simulink model "WTmodel"  (R2016b)
settings: Solver=VariableStepAuto  StartTime=0.0  StopTime=10.0  RelTol=1e-3
values from neighbouring files (symbols this model uses):
  Kb = 56.6    [B2B_SM_wC_data_fromCC_WT.m]
undefined symbols (not defined in the file or in its folder): VPoptpu, wPrefpu
settings Model: Creator=peiyuan  LastModifiedBy=peiyuan

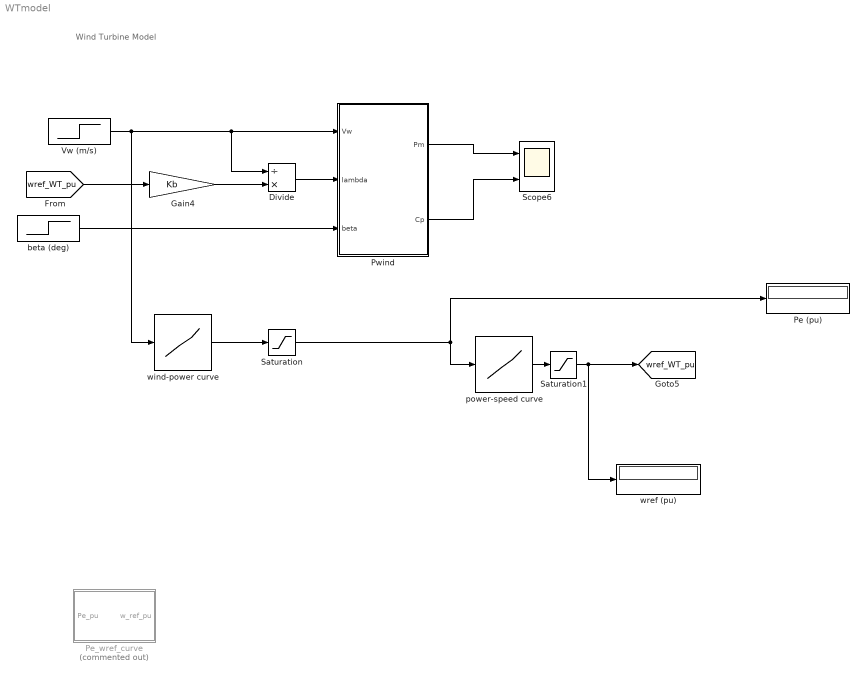
== system WTmodel ==
  note: Wind Turbine Model
  Divide : Product  Inputs=/*
  Gain4 : Gain  Gain=Kb
  Pe (pu) : Display
      settings: Format=bank
  Pe_wref_curve : Subsystem  Commented=on
  Pwind : MATLAB Function  TreatAsAtomicUnit=on
  Saturation : Saturate  UpperLimit=1  LowerLimit=0
  Saturation1 : Saturate  UpperLimit=1.2  LowerLimit=0.1
  Scope6 : Scope  NumInputPorts=2
  "Vw (m/s) " : Step  Time=5  Before=9  After=15  SampleTime=0
  beta (deg) : Step  Time=5  After=11.47  SampleTime=0
  power-speed curve : Lookup_n-D  NumberOfTableDimensions=1  BreakpointsForDimension1=wPrefpu(:,2)  Table=wPrefpu(:,1)  InternalRulePriority=Speed  RndMeth=Simplest  InputSameDT=on
  wind-power curve : Lookup_n-D  NumberOfTableDimensions=1  BreakpointsForDimension1=VPoptpu(:,1)  Table=VPoptpu(:,2)  InternalRulePriority=Speed  RndMeth=Simplest  InputSameDT=on
  wref (pu) : Display
      settings: Format=bank
  tag scope: wref_WT_pu=global
  wires:
  "Vw (m/s) "/1 -> wind-power curve/1, Pwind/1(Vw), Divide/1
  Divide/1 -> Pwind/2(lambda)
  Gain4/1 -> Divide/2
  beta (deg)/1 -> Pwind/3(beta)
  [wref_WT_pu] -> Gain4/1
  Pwind/1(Pm) -> Scope6/1
  Pwind/2(Cp) -> Scope6/2
  wind-power curve/1 -> Saturation/1
  power-speed curve/1 -> Saturation1/1
  Saturation/1 -> power-speed curve/1, Pe (pu)/1
  Saturation1/1 -> wref (pu)/1, [wref_WT_pu]

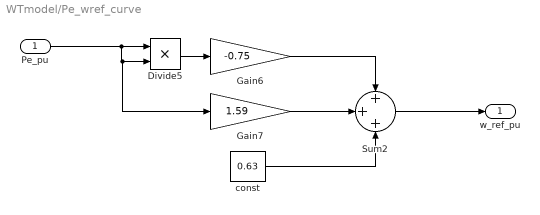
== system WTmodel/Pe_wref_curve ==
  Pe_pu : Inport
  Divide5 : Product  Inputs=**
  Gain6 : Gain  Gain=-0.75
  Gain7 : Gain  Gain=1.59
  Sum2 : Sum  Inputs=+++
  const : Constant  Value=0.63
  w_ref_pu : Outport
  wires:
  Gain7/1 -> Sum2/2
  Gain6/1 -> Sum2/1
  Divide5/1 -> Gain6/1
  Pe_pu/1 -> Gain7/1, Divide5/2, Divide5/1
  const/1 -> Sum2/3
  Sum2/1 -> w_ref_pu/1

== matlab function WTmodel/Pwind ==
  data: Vw input; Pm output; lambda input; beta input; Cp output
function [Pm,Cp] = Pwind(Vw,lambda,beta)

%% Inputs
% Vm
% beta: Pitch angle
% lambda: Tip speed ratio

%% Outputs
% Pm: Mechanical power output
% Cp: aerodynamic efficiency

%% Cp calculation: valid for lambda within (3,15)

alpha=[-4.1909e-1  2.1808e-1  -1.2406e-2  -1.3365e-4   1.1524e-5
       -6.7606e-2  6.0405e-2  -1.3934e-2   1.0683e-3  -2.3895e-5
        1.5727e-2 -1.0996e-2   2.1495e-3  -1.4855e-4   2.7937e-6
       -8.6018e-4  5.7051e-4  -1.0479e-4   5.9924e-6  -8.9194e-8
        1.4787e-5 -9.4839e-6   1.6167e-6  -7.1535e-8   4.9686e-10];

% Size of alpha
sz=size(alpha);
rw=sz(1);
cl=sz(2);

% calculate Cp
y=0;

for kk=1:rw
    
    for jj=1:cl
        
        y=y+alpha(kk,jj)*(beta^(kk-1))*(lambda^(jj-1));
        
    end
end
% Cp=min(max(y,-0.05),0.5173);
Cp=max(y,-0.05);

% GE 3.6 MW turbine mechanical power output
Ka=0.00159; % kg/m, 1/2*rho*Ar, defined directly inside function 'Pwind'
Pm = Ka*(Vw^3)*Cp;
